simulink library "lib_rfsoc_fec"  (R2020b)
settings: Solver=VariableStepAuto  StartTime=0.0  StopTime=10.0  RelTol=1e-3
undefined symbols (not defined in the file): d, fs, generator_polynomial
libraries: commseqgen3 x84, hdlsllib x83, $bdroot x33, simulink x22, dspsigops x13
(part 1 of 4)
settings Model: Creator=ckb13136  LastModifiedBy=ckb13136

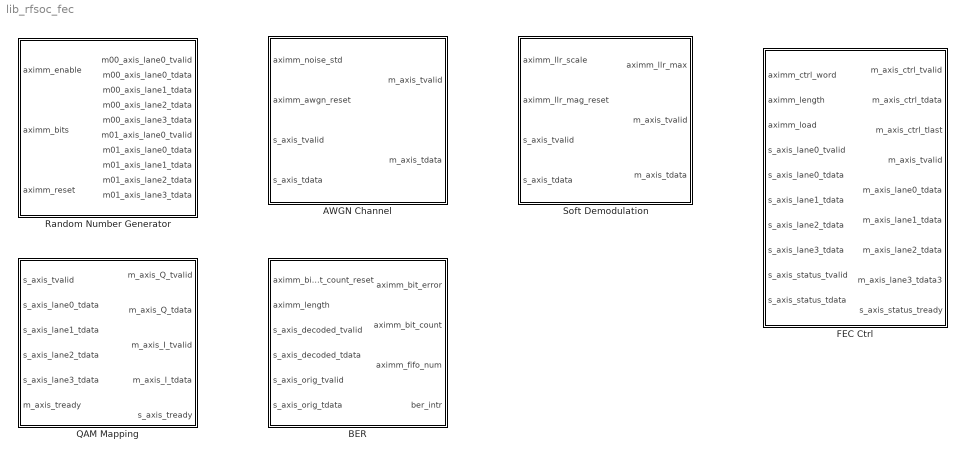
== system lib_rfsoc_fec ==
  AWGN Channel : Subsystem  TreatAsAtomicUnit=on
  BER : Subsystem  TreatAsAtomicUnit=on
  FEC Ctrl : Subsystem  TreatAsAtomicUnit=on
  QAM Mapping : Subsystem  TreatAsAtomicUnit=on
  Random Number Generator : Subsystem  TreatAsAtomicUnit=on
  Soft Demodulation : Subsystem  TreatAsAtomicUnit=on

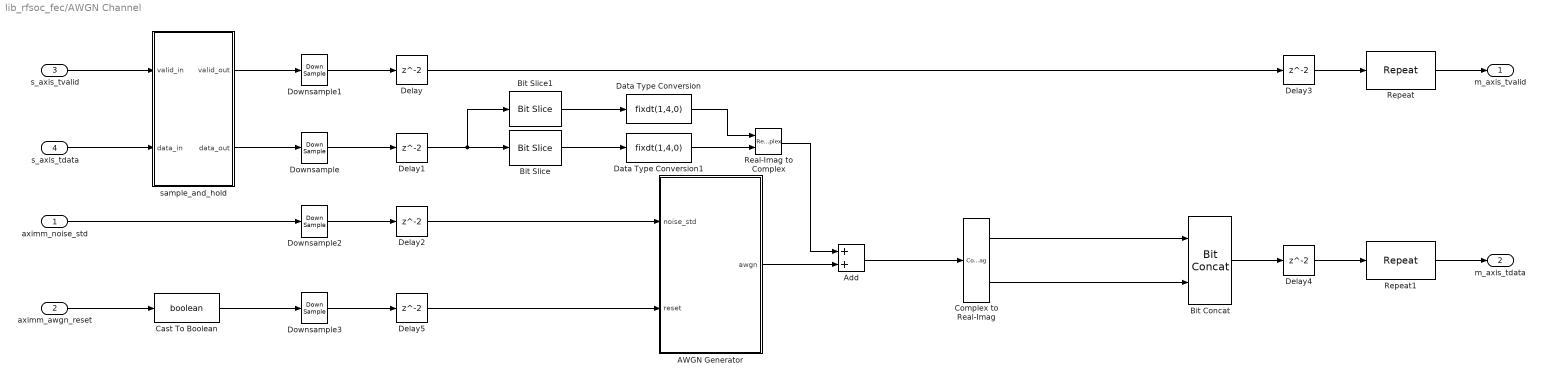
== system lib_rfsoc_fec/AWGN Channel ==
  aximm_noise_std : Inport
  aximm_awgn_reset : Inport  Port=2
  s_axis_tvalid : Inport  Port=3
  s_axis_tdata : Inport  Port=4
  AWGN Generator : Subsystem
  Add : Sum  OutDataTypeStr=fixdt(1,16,11)  SaturateOnIntegerOverflow=on
  Bit Concat : hdlsllib/Logic and Bit Operations/Bit Concat  numInputs=2
  Bit Slice : hdlsllib/Logic and Bit Operations/Bit Slice  lidx=3  ridx=0
      settings: SourceProductBaseCode=SL
  Bit Slice1 : hdlsllib/Logic and Bit Operations/Bit Slice  lidx=7  ridx=4
      settings: SourceProductBaseCode=SL
  Cast To Boolean : DataTypeConversion  OutDataTypeStr=boolean
  Complex to Real-Imag : ComplexToRealImag
  Data Type Conversion : DataTypeConversion  OutDataTypeStr=fixdt(1,4,0)  ConvertRealWorld=Stored Integer (SI)
  Data Type Conversion1 : DataTypeConversion  OutDataTypeStr=fixdt(1,4,0)  ConvertRealWorld=Stored Integer (SI)
  Delay{,1..5} (6 alike) : Delay
  Downsample{,1..3} (4 alike) : DownSample  N=4  RateOptions=Allow multirate processing
  Real-Imag to Complex : RealImagToComplex
  Repeat : dspsigops/Repeat  N=4  InputProcessing=Columns as channels (frame based)  RateOptions=Allow multirate processing  ic=0  mode=Unused parameter value
      settings: SourceProductName=DSP System Toolbox
  Repeat1 : dspsigops/Repeat  N=4  InputProcessing=Columns as channels (frame based)  RateOptions=Allow multirate processing  ic=0  mode=Unused parameter value
      settings: SourceProductName=DSP System Toolbox
  sample_and_hold : Subsystem
  m_axis_tvalid : Outport
  m_axis_tdata : Outport  Port=2
  wires:
  AWGN Generator/1(awgn) -> Add/2
  aximm_noise_std/1 -> Downsample2/1
  Delay2/1 -> AWGN Generator/1(noise_std)
  Downsample2/1 -> Delay2/1
  Delay5/1 -> AWGN Generator/2(reset)
  sample_and_hold/1(" valid_out") -> Downsample1/1
  Downsample1/1 -> Delay/1
  Downsample/1 -> Delay1/1
  Delay/1 -> Delay3/1
  sample_and_hold/2(" data_out") -> Downsample/1
  s_axis_tvalid/1 -> sample_and_hold/1(valid_in)
  s_axis_tdata/1 -> sample_and_hold/2(data_in)
  Delay1/1 -> Bit Slice1/1, Bit Slice/1
  Repeat1/1 -> m_axis_tdata/1
  Repeat/1 -> m_axis_tvalid/1
  Delay3/1 -> Repeat/1
  Delay4/1 -> Repeat1/1
  Bit Slice1/1 -> Data Type Conversion/1
  Bit Slice/1 -> Data Type Conversion1/1
  Data Type Conversion/1 -> Real-Imag to Complex/1
  Data Type Conversion1/1 -> Real-Imag to Complex/2
  Real-Imag to Complex/1 -> Add/1
  Add/1 -> Complex to Real-Imag/1
  Bit Concat/1 -> Delay4/1
  Complex to Real-Imag/1 -> Bit Concat/1
  Complex to Real-Imag/2 -> Bit Concat/2
  Downsample3/1 -> Delay5/1
  aximm_awgn_reset/1 -> Cast To Boolean/1
  Cast To Boolean/1 -> Downsample3/1

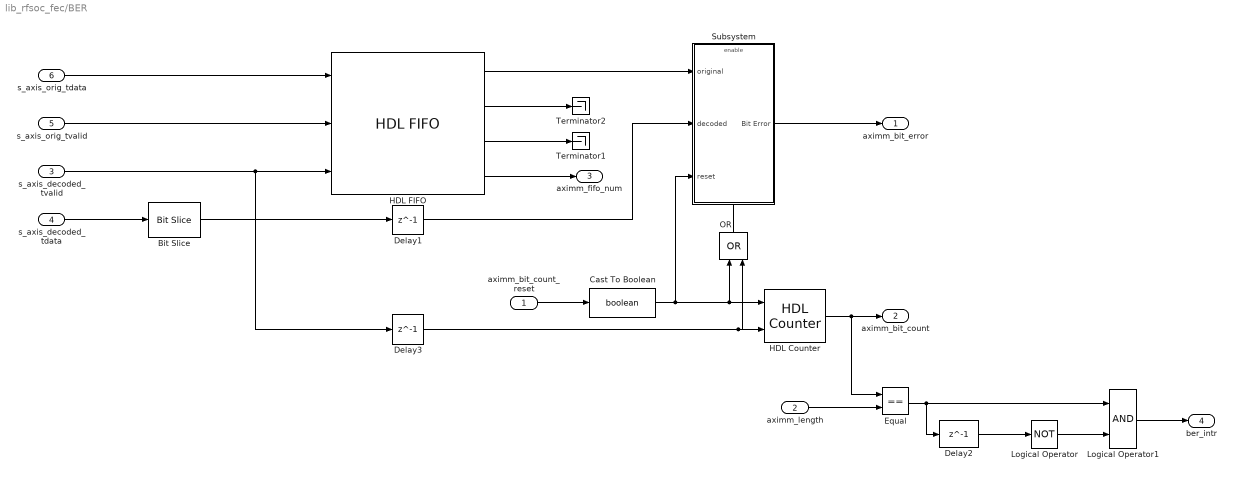
== system lib_rfsoc_fec/BER ==
  aximm_bit_count_reset : Inport
  aximm_length : Inport  Port=2
  s_axis_decoded_tvalid : Inport  Port=3
  s_axis_decoded_tdata : Inport  Port=4
  s_axis_orig_tvalid : Inport  Port=5
  s_axis_orig_tdata : Inport  Port=6
  Bit Slice : hdlsllib/Logic and Bit Operations/Bit Slice  lidx=7  ridx=0
      settings: SourceProductBaseCode=SL
  Cast To Boolean : DataTypeConversion  OutDataTypeStr=boolean
  Delay1 : Delay  DelayLength=1
  Delay2 : Delay  DelayLength=1  InitialCondition=1  InputProcessing=Columns as channels (frame based)
  Delay3 : Delay  DelayLength=1
  Equal : RelationalOperator  Operator===  OutDataTypeStr=boolean  RndMeth=Simplest
  HDL Counter : hdlsllib/Sources/HDL Counter  CountType=Free running  CountInit=0  CountStep=8  CountMax=25  CountFromType=Initial value  CountFrom=0  CountResetPort=on  CountLoadPort=off  CountEnbPort=on  CountDirPort=off  CountDataType=Unsigned  CountWordLen=32  CountFracLen=0  CountSampTime=1
  HDL FIFO : hdlsllib/HDL RAMs/HDL FIFO  fifo_size=8192  mode=Classic  ratio=1  push_msg=Warning  pop_msg=Warning  show_empty=on  show_full=on  show_num=on  LabelModeActiveChoice_Mode=Classic
      settings: SourceProductBaseCode=SL
  Logical Operator : Logic  Operator=NOT  Inputs=1
  Logical Operator1 : Logic
  OR : Logic  Operator=OR  IconShape=distinctive  AllPortsSameDT=off  OutDataTypeStr=boolean
  Subsystem : Subsystem
  Terminator1 : Terminator
  Terminator2 : Terminator
  aximm_bit_error : Outport
  aximm_bit_count : Outport  Port=2
  aximm_fifo_num : Outport  Port=3
  ber_intr : Outport  Port=4
  wires:
  HDL FIFO/4 -> aximm_fifo_num/1
  s_axis_decoded_tvalid/1 -> HDL FIFO/3, Delay3/1
  Delay3/1 -> OR/2, HDL Counter/2
  s_axis_decoded_tdata/1 -> Bit Slice/1
  s_axis_orig_tvalid/1 -> HDL FIFO/2
  HDL FIFO/3 -> Terminator1/1
  Subsystem/1(Bit Error) -> aximm_bit_error/1
  HDL FIFO/1 -> Subsystem/1(original)
  Delay1/1 -> Subsystem/2(decoded)
  HDL Counter/1 -> Equal/1, aximm_bit_count/1
  Bit Slice/1 -> Delay1/1
  s_axis_orig_tdata/1 -> HDL FIFO/1
  aximm_bit_count_reset/1 -> Cast To Boolean/1
  Cast To Boolean/1 -> OR/1, HDL Counter/1, Subsystem/3(reset)
  OR/1 -> Subsystem/Enable
  Logical Operator/1 -> Logical Operator1/2
  HDL FIFO/2 -> Terminator2/1
  Delay2/1 -> Logical Operator/1
  Logical Operator1/1 -> ber_intr/1
  Equal/1 -> Delay2/1, Logical Operator1/1
  aximm_length/1 -> Equal/2

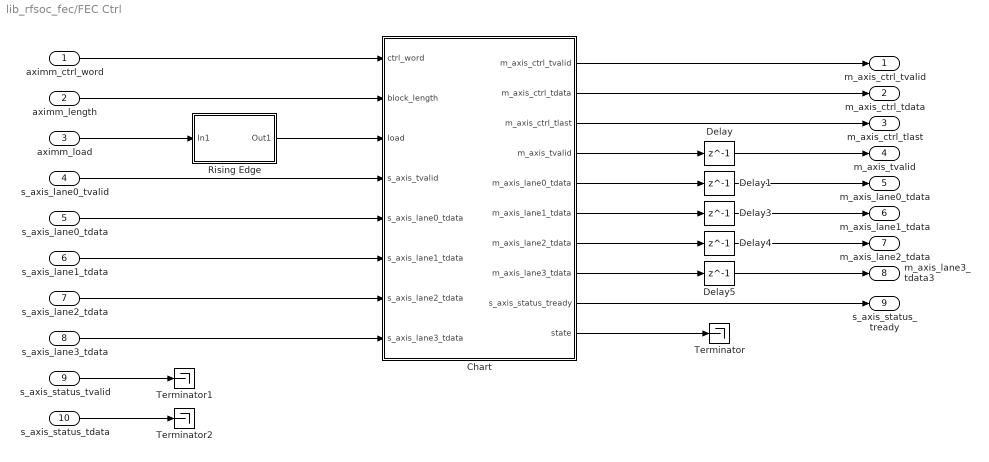
== system lib_rfsoc_fec/FEC Ctrl ==
  aximm_ctrl_word : Inport
  aximm_length : Inport  Port=2
  aximm_load : Inport  Port=3
  s_axis_lane0_tvalid : Inport  Port=4
  s_axis_lane0_tdata : Inport  Port=5
  s_axis_lane1_tdata : Inport  Port=6
  s_axis_lane2_tdata : Inport  Port=7
  s_axis_lane3_tdata : Inport  Port=8
  s_axis_status_tvalid : Inport  Port=9
  s_axis_status_tdata : Inport  Port=10
  Chart : Stateflow chart  TreatAsAtomicUnit=on
      settings: PortSchema="{\"entries\":[{\"content\":{\"sides\":[{\"content\":{\"connectorIds\":[\"In1\",\"In2\",\"In3\",\"In4\",\"In8\",\"In5\",\"In6\",\"In7\"]},\"type\":\"ConnectorPlacement.EquallySpacedRectSide\",\"uuid\":\"96b1e0a6-9243-45af-ad4c-9b6bdb766973\"},{\"content\":{\"connectorIds\":[\"Out1\",\"Out2\",\"Out3\",\"Out4\",\"Out7\",\"Out8\",\"Out9\",\"Out10\",\"Out5\",\"Out6\"],\"side\":\"RIGHT\"},\"type\":\"ConnectorPlacement.EquallySpacedRectSide\",\"uuid\":\"a962d190-29ee-4ef5-b85e-0d462d6476b7\"},{\"content\":{\"connectorIds\":[],\"side\":\"TOP\"},\"type\":\"ConnectorPlacement.EquallySpacedRectSide\",\"uuid\":\"6028541f-0eff-4bfb-a496-920287fbe05d\"},{\"content\":{\"connectorIds\":[],\"side\":\"HIDDEN\"},\"type\":\"ConnectorPlacement.EquallySpacedRectSide\",\"uuid\":\"2bd272f9-f96d-47a2-bf8a-d251a31e3228\"}]},\"type\":\"ConnectorPlacement.EquallySpacedConnector\",\"uuid\":\"9912cff3-58c1-4038-915e-716fff51edba\"}],\"packageUris\":[\"http://schema.mathworks.com/mf0/Connector/R2020b\"],\"version\":\"1.0\"}"
  Delay{,1,3..5} (5 alike) : Delay  DelayLength=1
  Rising Edge : Subsystem
  Terminator : Terminator
  Terminator1 : Terminator
  Terminator2 : Terminator
  m_axis_ctrl_tvalid : Outport
  m_axis_ctrl_tdata : Outport  Port=2
  m_axis_ctrl_tlast : Outport  Port=3
  m_axis_tvalid : Outport  Port=4
  m_axis_lane0_tdata : Outport  Port=5
  m_axis_lane1_tdata : Outport  Port=6
  m_axis_lane2_tdata : Outport  Port=7
  m_axis_lane3_tdata3 : Outport  Port=8
  s_axis_status_tready : Outport  Port=9
  wires:
  Chart/3(m_axis_ctrl_tlast) -> m_axis_ctrl_tlast/1
  Chart/6(state) -> Terminator/1
  aximm_length/1 -> Chart/2(block_length)
  s_axis_lane0_tvalid/1 -> Chart/4(s_axis_tvalid)
  s_axis_lane0_tdata/1 -> Chart/8(s_axis_lane0_tdata)
  aximm_ctrl_word/1 -> Chart/1(ctrl_word)
  Chart/2(m_axis_ctrl_tdata) -> m_axis_ctrl_tdata/1
  Chart/4(m_axis_tvalid) -> Delay/1
  Chart/5(s_axis_status_tready) -> s_axis_status_tready/1
  Chart/1(m_axis_ctrl_tvalid) -> m_axis_ctrl_tvalid/1
  Delay/1 -> m_axis_tvalid/1
  s_axis_status_tvalid/1 -> Terminator1/1
  s_axis_status_tdata/1 -> Terminator2/1
  Chart/8(m_axis_lane1_tdata) -> Delay3/1
  Chart/7(m_axis_lane0_tdata) -> Delay1/1
  Chart/9(m_axis_lane2_tdata) -> Delay4/1
  Chart/10(m_axis_lane3_tdata) -> Delay5/1
  Delay1/1 -> m_axis_lane0_tdata/1
  Delay5/1 -> m_axis_lane3_tdata3/1
  Delay4/1 -> m_axis_lane2_tdata/1
  Delay3/1 -> m_axis_lane1_tdata/1
  s_axis_lane1_tdata/1 -> Chart/5(s_axis_lane1_tdata)
  s_axis_lane2_tdata/1 -> Chart/6(s_axis_lane2_tdata)
  s_axis_lane3_tdata/1 -> Chart/7(s_axis_lane3_tdata)
  aximm_load/1 -> Rising Edge/1(In1)
  Rising Edge/1(Out1) -> Chart/3(load)

== system lib_rfsoc_fec/QAM Mapping ==
  s_axis_tvalid : Inport
  s_axis_lane0_tdata : Inport  Port=2
  s_axis_lane1_tdata : Inport  Port=3
  s_axis_lane2_tdata : Inport  Port=4
  s_axis_lane3_tdata : Inport  Port=5
  m_axis_tready : Inport  Port=6
  Buffer : Subsystem
  HDL Counter1 : hdlsllib/Sources/HDL Counter  CountType=Count limited  CountInit=0  CountStep=1  CountMax=3  CountFromType=Initial value  CountFrom=0  CountResetPort=off  CountLoadPort=off  CountEnbPort=on  CountDirPort=off  CountDataType=Unsigned  CountWordLen=2  CountFracLen=0  CountSampTime=1/(fs*2)
  Multiport Switch1 : MultiPortSwitch  DataPortOrder=Zero-based contiguous  Inputs=4  zeroidx=on
  QAM Mapping : Subsystem
  Terminator : Terminator
  m_axis_Q_tvalid : Outport
  m_axis_Q_tdata : Outport  Port=2
  m_axis_I_tvalid : Outport  Port=3
  m_axis_I_tdata : Outport  Port=4
  s_axis_tready : Outport  Port=5
  wires:
  QAM Mapping/2(I symbols) -> m_axis_I_tdata/1
  Multiport Switch1/1 -> QAM Mapping/1(bits lane0)
  HDL Counter1/1 -> Multiport Switch1/1
  Buffer/5(" lane3") -> Multiport Switch1/5
  Buffer/4(" lane2") -> Multiport Switch1/4
  Buffer/3(" lane1") -> Multiport Switch1/3
  Buffer/2(" lane0") -> Multiport Switch1/2
  Buffer/1(" valid_out") -> HDL Counter1/1, m_axis_Q_tvalid/1, m_axis_I_tvalid/1, QAM Mapping/Enable
  QAM Mapping/1(Q symbols) -> m_axis_Q_tdata/1
  m_axis_tready/1 -> Terminator/1
  s_axis_lane0_tdata/1 -> Buffer/2(s_axis_lane0_tdata)
  s_axis_tvalid/1 -> Buffer/1(s_axis_tvalid)
  s_axis_lane1_tdata/1 -> Buffer/3(s_axis_lane1_tdata)
  s_axis_lane2_tdata/1 -> Buffer/4(s_axis_lane2_tdata)
  s_axis_lane3_tdata/1 -> Buffer/5(s_axis_lane3_tdata)
  Buffer/6(s_axis_tready) -> s_axis_tready/1

== system lib_rfsoc_fec/Random Number Generator ==
  aximm_enable : Inport
  aximm_bits : Inport  Port=2
  aximm_reset : Inport  Port=3
  Cast To Boolean1 : DataTypeConversion  OutDataTypeStr=boolean
  Random Number Generator : Subsystem  mask{bits=64, gen_poly=generator_polynomial}
      mask prompts: bits "Data Bits:"; gen_poly "Generator Polynomial:"
      mask init:
      | random_gen = gcb;
      | 
      | %set_param(random_gen, 'LinkStatus', 'none');
      | 
      | block_handles = Simulink.findBlocks(gcb);
      | block_names = getfullname(block_handles);
      | 
      | out_block = sprintf('%s/data', random_gen);
      | in_block = sprintf('%s/reset', random_gen);
      | enable_block = sprintf('%s/enable', random_gen);
      | 
      | keep_blocks = {out_block, in_block, enable_block};
      | 
      | for i = 1:length(block_names)
      |     if ~ismember(block_names{i}, keep_blocks)
      |         delete_block(block_names{i});
      |     end
      | end
      | delete_line(find_system(random_gen,'LookUnderMasks', 'all','FindAll','on','type','line'));
      | 
      | % Add all PN Sequence Generators 
      | for bit = 1:bits
      |     current_block = sprintf('%s/bit%d', random_gen, bit-1);
      |     add_block('commseqgen3/PN Sequence Generator', current_block);
      |     position = get_param(current_block, 'position');
      |     if bit == 1
      |         start_position = position;
      |     end
      |     new_position = position + ([0 60 0 60] * (bit-1));
      |     set_param(current_block, 'position', new_position);
      |     set_param(current_block, 'outDataType', 'boolean');
      |     set_param(current_block, 'reset', 'on');
      |     set_param(current_block, 'Ts', '-1');
      |     set_param(current_block, 'poly', gen_poly);
      |     
      |     val = dec2bin(randi(2^13 - 1), 13);
      |     str = '[';
      |     for i = 1:13
      |         str(end+1:end+2) = [' ' (val(i))];
      |     end
      |     str(end+1) = ']';
      |     set_param(current_block, 'ini_sta', str);
      | end
      | 
      | % Add the Bit Concat
      | concat_block = sprintf('%s/concat', random_gen);
      | add_block('hdlsllib/Logic and Bit Operations/Bit Concat', concat_block);
      | set_param(concat_block, 'numInputs', num2str(bits));
      | position = new_position + [150 0 150 0];
      | position(2) = start_position(2);
      | set_param(concat_block, 'position', position);
      | 
      | % Add Input and Outputs
      | out_position = get_param(out_block, 'position');
      | height = out_position(4) - out_position(2);
      | width = out_position(3) - out_position(1);
      | middle_h = (position(4) - position(2))/2 + position(2);
      | out_position = [position(1) + 150, middle_h - height/2, position(1) + 150 + width, middle_h + height/2];
      | set_param(out_block, 'position', out_position);
      | 
      | in_position = [position(1) - 300, middle_h - height/2, position(1) - 300 + width, middle_h + height/2];
      | set_param(in_block, 'position', in_position);
      | 
      | enable_position = get_param(enable_block, 'position');
      | set_param(enable_block, 'position', enable_position - [0 100 0 100]);
      | 
      | % Connect Ports
      | for bit = 1:bits
      |     add_line(random_gen,'reset/1', sprintf('bit%d/1', bit-1));
      |     add_line(random_gen,sprintf('bit%d/1', bit-1), sprintf('concat/%d', bit));
      | end
      | add_line(random_gen,'concat/1','data/1');
      mask DialogControl DescGroupVar Prompt: N-Bit Random Number Generator
      mask DialogControl DescTextVar Prompt: This block will create a n-bit random number generator. Provide a polynomial and the number of bits. Information on polynomials for maximal LFSRs can be found:  https://en.wikipedia.org/wiki/Linear-feedback_shift_register For example: ''z^13 + z^12 + z^11 + z^8 + 1''
  Terminator : Terminator
  Terminator1 : Terminator
  Terminator2 : Terminator
  byte_count : Subsystem
  concat : Subsystem
  hold for multiple of 4 : Subsystem
  interface_creator : Subsystem
  rising_edge : Subsystem
  tvalid hold : Subsystem
  m00_axis_lane0_tvalid : Outport
  m00_axis_lane0_tdata : Outport  Port=2
  m00_axis_lane1_tdata : Outport  Port=3
  m00_axis_lane2_tdata : Outport  Port=4
  m00_axis_lane3_tdata : Outport  Port=5
  m01_axis_lane0_tvalid : Outport  Port=6
  m01_axis_lane0_tdata : Outport  Port=7
  m01_axis_lane1_tdata : Outport  Port=8
  m01_axis_lane2_tdata : Outport  Port=9
  m01_axis_lane3_tdata : Outport  Port=10
  wires:
  hold for multiple of 4/1(" ") -> byte_count/2(en)
  concat/1(d_out) -> interface_creator/3(data_in)
  interface_creator/7(lane_3_tvalid) -> Terminator2/1
  interface_creator/5(lane_2_tvalid) -> Terminator1/1
  interface_creator/3(lane_1_tvalid) -> Terminator/1
  Random Number Generator/1(data) -> concat/2(d_in)
  tvalid hold/2(diff) -> concat/3(diff)
  interface_creator/1(lane_0_tvalid) -> m00_axis_lane0_tvalid/1, m01_axis_lane0_tvalid/1
  byte_count/2(valid) -> interface_creator/2(en)
  byte_count/1(count) -> interface_creator/1(count)
  Cast To Boolean1/1 -> Random Number Generator/1(reset), byte_count/1(reset)
  tvalid hold/1(enable) -> hold for multiple of 4/1(In1), Random Number Generator/Enable, concat/1(en)
  aximm_bits/1 -> tvalid hold/2(comparator)
  rising_edge/1(pulse) -> tvalid hold/1(trigger)
  aximm_enable/1 -> rising_edge/1(in)
  aximm_reset/1 -> Cast To Boolean1/1
  interface_creator/2(lane_0_tdata) -> m00_axis_lane0_tdata/1, m01_axis_lane0_tdata/1
  interface_creator/6(lane_2_tdata) -> m01_axis_lane2_tdata/1, m00_axis_lane2_tdata/1
  interface_creator/8(lane_3_tdata) -> m01_axis_lane3_tdata/1, m00_axis_lane3_tdata/1
  interface_creator/4(lane_1_tdata) -> m01_axis_lane1_tdata/1, m00_axis_lane1_tdata/1

== system lib_rfsoc_fec/Soft Demodulation ==
  aximm_llr_scale : Inport
  aximm_llr_mag_reset : Inport  Port=2
  s_axis_tvalid : Inport  Port=3
  s_axis_tdata : Inport  Port=4
  Bit Slice : hdlsllib/Logic and Bit Operations/Bit Slice  lidx=15  ridx=0
      settings: SourceProductBaseCode=SL
  Bit Slice1 : hdlsllib/Logic and Bit Operations/Bit Slice  lidx=31  ridx=16
      settings: SourceProductBaseCode=SL
  Cast To Boolean : DataTypeConversion  OutDataTypeStr=boolean
  Data Type Conversion : DataTypeConversion  OutDataTypeStr=fixdt(1,16,11)  ConvertRealWorld=Stored Integer (SI)
  Data Type Conversion1 : DataTypeConversion  OutDataTypeStr=fixdt(1,16,11)  ConvertRealWorld=Stored Integer (SI)
  MATLAB Function : MATLAB Function  TreatAsAtomicUnit=on
  Soft Demodulation : Subsystem
  sign_extend : Subsystem
  symmetric_saturation : MATLAB Function  TreatAsAtomicUnit=on
  aximm_llr_max : Outport
  m_axis_tvalid : Outport  Port=2
  m_axis_tdata : Outport  Port=3
  wires:
  aximm_llr_scale/1 -> Soft Demodulation/4(LLR Scale)
  Soft Demodulation/1(LLR Values) -> symmetric_saturation/1(u), MATLAB Function/1(u)
  s_axis_tvalid/1 -> m_axis_tvalid/1, Soft Demodulation/1(valid)
  MATLAB Function/1(y) -> aximm_llr_max/1
  aximm_llr_mag_reset/1 -> Cast To Boolean/1
  sign_extend/1(y) -> m_axis_tdata/1
  symmetric_saturation/1(y) -> sign_extend/1(u)
  Cast To Boolean/1 -> MATLAB Function/2(reset)
  Bit Slice1/1 -> Data Type Conversion/1
  Bit Slice/1 -> Data Type Conversion1/1
  Data Type Conversion/1 -> Soft Demodulation/2(real)
  s_axis_tdata/1 -> Bit Slice1/1, Bit Slice/1
  Data Type Conversion1/1 -> Soft Demodulation/3(imag)

== system lib_rfsoc_fec/AWGN Channel/AWGN Generator ==
  noise_std : Inport
  reset : Inport  Port=2
  1-D Lookup Table : Lookup_n-D  NumberOfTableDimensions=1  BreakpointsForDimension1=[0:4095]  BreakpointsForDimension1DataTypeStr=fixdt(0,12,0)  IndexSearchMethod=Evenly spaced points  Table=d  InterpMethod=Flat  ExtrapMethod=Clip  DiagnosticForOutOfRangeInput=Error  InternalRulePriority=Speed  OutDataTypeStr=fixdt(1,18,14)  RndMeth=Simplest  InputSameDT=on
  Cosine Lookup : Lookup_n-D  NumberOfTableDimensions=1  BreakpointsForDimension1=[0:255]  IndexSearchMethod=Evenly spaced points  Table=cos([0:255]*2*pi/256)  InterpMethod=Flat  ExtrapMethod=Clip  DiagnosticForOutOfRangeInput=Error  UseLastTableValue=on  OutDataTypeStr=fixdt(1,16,14)  RndMeth=Simplest  InputSameDT=on
  Data Type Conversion : DataTypeConversion  OutDataTypeStr=fixdt(0,16,14)  RndMeth=Round  SaturateOnIntegerOverflow=on
  Gain : Gain  Gain=0.7  OutDataTypeStr=fixdt(1,15,11)  RndMeth=Nearest  SaturateOnIntegerOverflow=on
  Product : Product  OutDataTypeStr=fixdt(1,17,14)  RndMeth=Round  SaturateOnIntegerOverflow=on
  Product1 : Product  OutDataTypeStr=fixdt(1,17,14)  RndMeth=Round  SaturateOnIntegerOverflow=on
  Product3 : Product  OutDataTypeStr=fixdt(1,18,14)  RndMeth=Round
  Real-Imag to Complex1 : RealImagToComplex
  Sine Lookup : Lookup_n-D  NumberOfTableDimensions=1  BreakpointsForDimension1=[0:255]  IndexSearchMethod=Evenly spaced points  Table=sin([0:255]*2*pi/256)  InterpMethod=Flat  ExtrapMethod=Clip  DiagnosticForOutOfRangeInput=Error  UseLastTableValue=on  OutDataTypeStr=fixdt(1,16,14)  RndMeth=Simplest  InputSameDT=on
  Subsystem3 : Subsystem
  awgn : Outport
  wires:
  noise_std/1 -> Data Type Conversion/1
  Product1/1 -> Real-Imag to Complex1/1
  Product/1 -> Real-Imag to Complex1/2
  Product3/1 -> Gain/1
  Sine Lookup/1 -> Product/1
  reset/1 -> Subsystem3/1(Reset)
  Subsystem3/2(LFSR_F) -> 1-D Lookup Table/1
  1-D Lookup Table/1 -> Product1/2, Product/2
  Subsystem3/1(LFSR_G) -> Cosine Lookup/1, Sine Lookup/1
  Cosine Lookup/1 -> Product1/1
  Gain/1 -> awgn/1
  Real-Imag to Complex1/1 -> Product3/2
  Data Type Conversion/1 -> Product3/1

== system lib_rfsoc_fec/AWGN Channel/sample_and_hold ==
  valid_in : Inport
  data_in : Inport  Port=2
  Sample and Hold : dspsigops/Sample and Hold  trig=Rising edge  initCond=0  latchinput=off
  tvalid hold : Subsystem
  " valid_out" : Outport
  " data_out" : Outport  Port=2
  wires:
  valid_in/1 -> tvalid hold/1(In1), Sample and Hold/Trigger
  tvalid hold/1(" ") -> " valid_out"/1
  data_in/1 -> Sample and Hold/1
  Sample and Hold/1 -> " data_out"/1

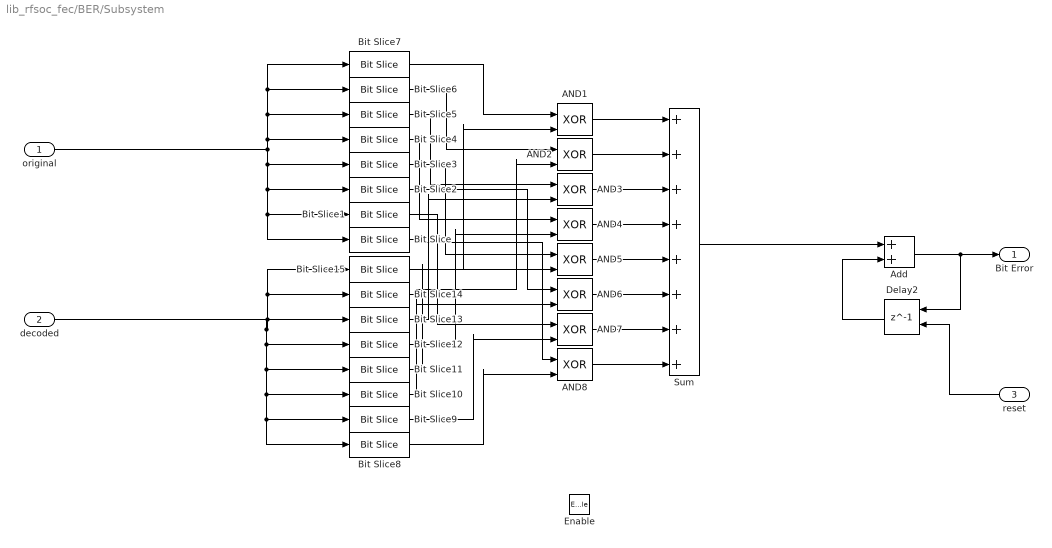
== system lib_rfsoc_fec/BER/Subsystem ==
  original : Inport
  decoded : Inport  Port=2
  reset : Inport  Port=3
  Enable : EnablePort
  AND{1..8} (8 alike) : Logic  Operator=XOR  IconShape=distinctive  AllPortsSameDT=off  OutDataTypeStr=boolean
  Add : Sum  OutDataTypeStr=uint32
  Bit Slice : hdlsllib/Logic and Bit Operations/Bit Slice  lidx=0  ridx=0
      settings: SourceProductBaseCode=SL
  Bit Slice1 : hdlsllib/Logic and Bit Operations/Bit Slice  lidx=1  ridx=1
      settings: SourceProductBaseCode=SL
  Bit Slice10 : hdlsllib/Logic and Bit Operations/Bit Slice  lidx=2  ridx=2
      settings: SourceProductBaseCode=SL
  Bit Slice11 : hdlsllib/Logic and Bit Operations/Bit Slice  lidx=3  ridx=3
      settings: SourceProductBaseCode=SL
  Bit Slice12 : hdlsllib/Logic and Bit Operations/Bit Slice  lidx=4  ridx=4
      settings: SourceProductBaseCode=SL
  Bit Slice13 : hdlsllib/Logic and Bit Operations/Bit Slice  lidx=5  ridx=5
      settings: SourceProductBaseCode=SL
  Bit Slice14 : hdlsllib/Logic and Bit Operations/Bit Slice  lidx=6  ridx=6
      settings: SourceProductBaseCode=SL
  Bit Slice15 : hdlsllib/Logic and Bit Operations/Bit Slice  lidx=7  ridx=7
      settings: SourceProductBaseCode=SL
  Bit Slice2 : hdlsllib/Logic and Bit Operations/Bit Slice  lidx=2  ridx=2
      settings: SourceProductBaseCode=SL
  Bit Slice3 : hdlsllib/Logic and Bit Operations/Bit Slice  lidx=3  ridx=3
      settings: SourceProductBaseCode=SL
  Bit Slice4 : hdlsllib/Logic and Bit Operations/Bit Slice  lidx=4  ridx=4
      settings: SourceProductBaseCode=SL
  Bit Slice5 : hdlsllib/Logic and Bit Operations/Bit Slice  lidx=5  ridx=5
      settings: SourceProductBaseCode=SL
  Bit Slice6 : hdlsllib/Logic and Bit Operations/Bit Slice  lidx=6  ridx=6
      settings: SourceProductBaseCode=SL
  Bit Slice7 : hdlsllib/Logic and Bit Operations/Bit Slice  lidx=7  ridx=7
      settings: SourceProductBaseCode=SL
  Bit Slice8 : hdlsllib/Logic and Bit Operations/Bit Slice  lidx=0  ridx=0
      settings: SourceProductBaseCode=SL
  Bit Slice9 : hdlsllib/Logic and Bit Operations/Bit Slice  lidx=1  ridx=1
      settings: SourceProductBaseCode=SL
  Delay2 : Delay  DelayLength=1  ExternalReset=Level
      settings: InputPortMap=u0,r5
  Sum : Sum  Inputs=++++++++  OutDataTypeStr=fixdt(0,3,0)  SaturateOnIntegerOverflow=on
  Bit Error : Outport  InitialOutput=0
  wires:
  Bit Slice14/1 -> AND2/2
  original/1 -> Bit Slice/1, Bit Slice1/1, Bit Slice2/1, Bit Slice3/1, Bit Slice4/1, Bit Slice5/1, Bit Slice6/1, Bit Slice7/1
  AND5/1 -> Sum/5
  Delay2/1 -> Add/2
  Bit Slice15/1 -> AND1/2
  AND2/1 -> Sum/2
  Bit Slice6/1 -> AND2/1
  AND4/1 -> Sum/4
  decoded/1 -> Bit Slice8/1, Bit Slice9/1, Bit Slice10/1, Bit Slice11/1, Bit Slice12/1, Bit Slice13/1, Bit Slice15/1, Bit Slice14/1
  AND6/1 -> Sum/6
  Sum/1 -> Add/1
  AND7/1 -> Sum/7
  Bit Slice2/1 -> AND6/1
  AND8/1 -> Sum/8
  Bit Slice/1 -> AND8/1
  Bit Slice4/1 -> AND4/1
  Bit Slice3/1 -> AND5/1
  Bit Slice5/1 -> AND3/1
  Bit Slice7/1 -> AND1/1
  Bit Slice8/1 -> AND8/2
  Add/1 -> Bit Error/1, Delay2/1
  Bit Slice10/1 -> AND6/2
  Bit Slice12/1 -> AND4/2
  Bit Slice9/1 -> AND7/2
  Bit Slice1/1 -> AND7/1
  AND3/1 -> Sum/3
  Bit Slice13/1 -> AND3/2
  Bit Slice11/1 -> AND5/2
  AND1/1 -> Sum/1
  reset/1 -> Delay2/2

== system lib_rfsoc_fec/FEC Ctrl/Rising Edge ==
  In1 : Inport
  Data Type Conversion1 : DataTypeConversion  OutDataTypeStr=boolean  SaturateOnIntegerOverflow=on  RndMeth=Zero
  Delay2 : Delay  DelayLength=1  InitialCondition=1  InputProcessing=Columns as channels (frame based)
  Logical Operator : Logic  Operator=NOT  Inputs=1
  Logical Operator1 : Logic
  Out1 : Outport
  wires:
  Logical Operator1/1 -> Out1/1
  Delay2/1 -> Logical Operator/1
  Logical Operator/1 -> Logical Operator1/2
  Data Type Conversion1/1 -> Delay2/1, Logical Operator1/1
  In1/1 -> Data Type Conversion1/1

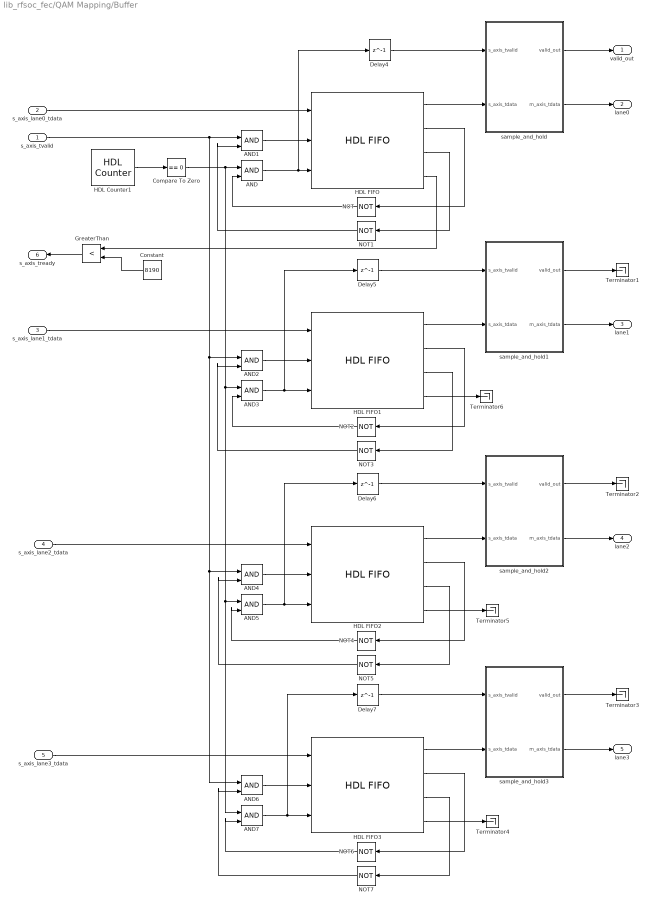
== system lib_rfsoc_fec/QAM Mapping/Buffer ==
  s_axis_tvalid : Inport
  s_axis_lane0_tdata : Inport  Port=2
  s_axis_lane1_tdata : Inport  Port=3
  s_axis_lane2_tdata : Inport  Port=4
  s_axis_lane3_tdata : Inport  Port=5
  AND{,1..7} (8 alike) : Logic  IconShape=distinctive  AllPortsSameDT=off  OutDataTypeStr=boolean
  Compare To Zero : simulink/Logic and Bit Operations/Compare To Zero  relop===  OutDataTypeStr=boolean
  Constant : Constant  Value=8190  OutDataTypeStr=fixdt(0,log2(8190),0)  SampleTime=1/(fs*2)
  Delay{4..7} (4 alike) : Delay  DelayLength=1
  GreaterThan : RelationalOperator  Operator=<  OutDataTypeStr=boolean  RndMeth=Simplest
  HDL Counter1 : hdlsllib/Sources/HDL Counter  CountType=Free running  CountInit=0  CountStep=1  CountMax=1  CountFromType=Initial value  CountFrom=0  CountResetPort=off  CountLoadPort=off  CountEnbPort=off  CountDirPort=off  CountDataType=Unsigned  CountWordLen=2  CountFracLen=0  CountSampTime=1/(fs*2)
  HDL FIFO{,1..3} (4 alike) : hdlsllib/HDL RAMs/HDL FIFO  fifo_size=128  mode=Classic  ratio=1  push_msg=Warning  pop_msg=Warning  show_empty=on  show_full=on  show_num=on  LabelModeActiveChoice_Mode=Classic
      settings: SourceProductBaseCode=SL
  NOT{,1..7} (8 alike) : Logic  Operator=NOT  IconShape=distinctive  AllPortsSameDT=off  OutDataTypeStr=boolean
  Terminator{1..6} (6 alike) : Terminator
  sample_and_hold : Subsystem
  sample_and_hold1 : Subsystem
  sample_and_hold2 : Subsystem
  sample_and_hold3 : Subsystem
  " valid_out" : Outport
  " lane0" : Outport  Port=2
  " lane1" : Outport  Port=3
  " lane2" : Outport  Port=4
  " lane3" : Outport  Port=5
  s_axis_tready : Outport  Port=6
  wires:
  sample_and_hold3/1(" valid_out") -> Terminator3/1
  sample_and_hold3/2(" m_axis_tdata") -> " lane3"/1
  sample_and_hold2/2(" m_axis_tdata") -> " lane2"/1
  sample_and_hold2/1(" valid_out") -> Terminator2/1
  AND/1 -> Delay4/1, HDL FIFO/3
  HDL FIFO/1 -> sample_and_hold/2(s_axis_tdata)
  NOT/1 -> AND/2
  AND7/1 -> Delay7/1, HDL FIFO3/3
  sample_and_hold1/1(" valid_out") -> Terminator1/1
  Compare To Zero/1 -> AND7/1, AND5/1, AND3/1, AND/1
  NOT5/1 -> AND4/2
  Delay4/1 -> sample_and_hold/1(s_axis_tvalid)
  HDL FIFO2/1 -> sample_and_hold2/2(s_axis_tdata)
  s_axis_lane0_tdata/1 -> HDL FIFO/1
  NOT4/1 -> AND5/2
  s_axis_tvalid/1 -> AND6/1, AND4/1, AND2/1, AND1/1
  AND5/1 -> Delay6/1, HDL FIFO2/3
  HDL FIFO1/1 -> sample_and_hold1/2(s_axis_tdata)
  HDL FIFO3/3 -> NOT7/1
  NOT7/1 -> AND6/2
  NOT1/1 -> AND1/2
  Constant/1 -> GreaterThan/2
  HDL FIFO2/4 -> Terminator5/1
  s_axis_lane3_tdata/1 -> HDL FIFO3/1
  HDL FIFO/3 -> NOT1/1
  s_axis_lane2_tdata/1 -> HDL FIFO2/1
  AND3/1 -> Delay5/1, HDL FIFO1/3
  s_axis_lane1_tdata/1 -> HDL FIFO1/1
  HDL Counter1/1 -> Compare To Zero/1
  AND1/1 -> HDL FIFO/2
  HDL FIFO3/4 -> Terminator4/1
  Delay7/1 -> sample_and_hold3/1(s_axis_tvalid)
  Delay6/1 -> sample_and_hold2/1(s_axis_tvalid)
  HDL FIFO1/3 -> NOT3/1
  HDL FIFO2/3 -> NOT5/1
  HDL FIFO3/2 -> NOT6/1
  HDL FIFO/4 -> GreaterThan/1
  HDL FIFO1/2 -> NOT2/1
  AND6/1 -> HDL FIFO3/2
  HDL FIFO/2 -> NOT/1
  NOT2/1 -> AND3/2
  NOT6/1 -> AND7/2
  HDL FIFO3/1 -> sample_and_hold3/2(s_axis_tdata)
  GreaterThan/1 -> s_axis_tready/1
  HDL FIFO2/2 -> NOT4/1
  AND4/1 -> HDL FIFO2/2
  NOT3/1 -> AND2/2
  AND2/1 -> HDL FIFO1/2
  Delay5/1 -> sample_and_hold1/1(s_axis_tvalid)
  sample_and_hold/1(" valid_out") -> " valid_out"/1
  HDL FIFO1/4 -> Terminator6/1
  sample_and_hold/2(" m_axis_tdata") -> " lane0"/1
  sample_and_hold1/2(" m_axis_tdata") -> " lane1"/1

== system lib_rfsoc_fec/QAM Mapping/QAM Mapping ==
  bits lane0 : Inport
  Enable : EnablePort
  N-Width QAM-16 Symbol Mapping Imag : Subsystem  mask{bits=128}
      mask prompts: bits "Width:"
      mask init:
      | top_block = gcb;
      | % set_param(top_block, 'LinkStatus', 'none');
      | 
      | block_names = find_system(top_block, 'LookUnderMasks','on', 'SearchDepth','1');
      | 
      | in_block = sprintf('%s/bits', top_block);
      | out_block = sprintf('%s/symbol', top_block);
      | qam_16_block = sprintf('%s/QAM-16 Symbol Mapping 0', top_block);
      | % enable_block = sprintf('%s/enable', n_qam_16);
      | 
      | keep_blocks = {top_block, in_block, out_block, qam_16_block};
      | 
      | for i = 1:length(block_names)
      |     if ~ismember(block_names{i}, keep_blocks)
      |         delete_block(block_names{i});
      |     end
      | end
      | delete_line(find_system(top_block,'LookUnderMasks', 'all','SearchDepth', '1', 'FindAll','on','type','line'));
      | 
      | % Add QAM-16 Mapping Blocks
      | pos = get_param(qam_16_block, 'position');
      | new_pos = pos;
      | set_param(qam_16_block, 'n', num2str(bits-4));
      | for bit = 4:4:bits-1
      |     new_block = sprintf('%s%d', qam_16_block(1:end-1), bit/4);
      |     add_block(qam_16_block, new_block);
      |     new_pos = pos + ([0 60 0 60] * (bit/4));
      |     set_param(new_block, 'position', new_pos);
      |     set_param(new_block, 'n', num2str(bits-4-bit));
      | end
      | 
      | % Add the Bit Concat
      | concat_block = sprintf('%s/concat', top_block);
      | add_block('hdlsllib/Logic and Bit Operations/Bit Concat', concat_block);
      | set_param(concat_block, 'numInputs', num2str(bits/4));
      | concat_position = new_pos + [175 0 175 0];
      | concat_position(2) = pos(2);
      | set_param(concat_block, 'position', concat_position);
      | 
      | % Reposition Input and Outputs
      | out_position = get_param(out_block, 'position');
      | height = out_position(4) - out_position(2);
      | width = out_position(3) - out_position(1);
      | middle_h = (concat_position(4) - concat_position(2))/2 + concat_position(2);
      | out_position = [concat_position(1) + 175, middle_h - height/2, concat_position(1) + 175 + width, middle_h + height/2];
      | set_param(out_block, 'position', out_position);
      | 
      | in_position = [concat_position(1) - 300, middle_h - height/2, concat_position(1) - 300 + width, middle_h + height/2];
      | set_param(in_block, 'position', in_position);
      | 
      | % enable_position = get_param(enable_block, 'position');
      | % set_param(enable_block, 'position', enable_position - [0 100 0 100]);
      | 
      | % Connect Ports
      | for bit = 1:4:bits
      |     add_line(top_block,'bits/1',sprintf('QAM-16 Symbol Mapping %d/1',(bit-1)/4));
      |     add_line(top_block,sprintf('QAM-16 Symbol Mapping %d/1',(bit-1)/4),sprintf('concat/%d', ceil(bit/4)));
      | %     add_line(top_block,sprintf('QAM-16 Symbol Mapping %d/2',(bit-1)/4),sprintf('concat/%d', ceil(bit/2)+1));
      | end
      | add_line(top_block,'concat/1','symbol/1');
  N-Width QAM-16 Symbol Mapping Real : Subsystem  mask{bits=128}
      mask prompts: bits "Width:"
      mask init: same as lib_rfsoc_fec/QAM Mapping/QAM Mapping/N-Width QAM-16 Symbol Mapping Imag
  Q symbols : Outport
  I symbols : Outport  Port=2
  wires:
  N-Width QAM-16 Symbol Mapping Imag/1(symbol) -> Q symbols/1
  N-Width QAM-16 Symbol Mapping Real/1(symbol) -> I symbols/1
  bits lane0/1 -> N-Width QAM-16 Symbol Mapping Real/1(bits), N-Width QAM-16 Symbol Mapping Imag/1(bits)
